simulink model "PuntoEquilibrio"  (R2015a)
settings: Solver=ode45  StartTime=0.0  StopTime=50  RelTol=1e-3
values from neighbouring files (symbols this model uses):
  b = 2.64e-4    (= 0.000264)    [ParametrosQuadcoptero.m]
  d = 7.5e-7    (= 7.5e-07)    [ParametrosQuadcoptero.m]
  g = 9.81    [ParametrosQuadcoptero.m]
  Ix = 0.033    [ParametrosQuadcoptero.m]
  Iy = 0.033    [ParametrosQuadcoptero.m]
  Iz = 0.066    [ParametrosQuadcoptero.m]
  L = 0.5    [ParametrosQuadcoptero.m]
  m = 4    [ParametrosQuadcoptero.m]
  sys = ss(A,B,C,D,Ts)    [ModeloVariablesEstado.m]
  Ts = 0.05    [ModeloVariablesEstado.m]
  x10_0 = 0    [CondicionesIniciales.m]
  x11_0 = 0    [CondicionesIniciales.m]
  x12_0 = 0    [CondicionesIniciales.m]
  x1_0 = 0    [CondicionesIniciales.m]
  x2_0 = 0    [CondicionesIniciales.m]
  x3_0 = 0    [CondicionesIniciales.m]
  x4_0 = 0    [CondicionesIniciales.m]
  x5_0 = 10    [CondicionesIniciales.m]
  x6_0 = 0    [CondicionesIniciales.m]
  x7_0 = 0    [CondicionesIniciales.m]
  x8_0 = 0    [CondicionesIniciales.m]
  x9_0 = 0    [CondicionesIniciales.m]
libraries: mpclib x1
settings Model: Creator=Dell  LastModifiedBy=Dell

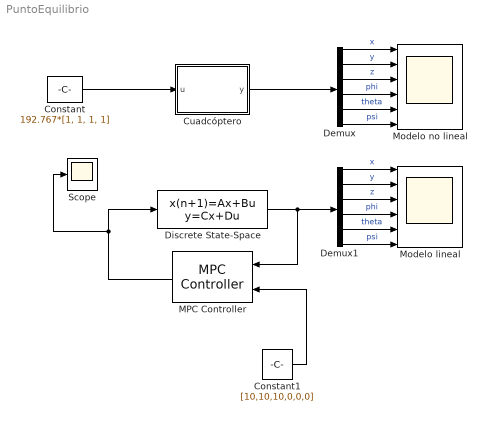
== system PuntoEquilibrio ==
  Constant : Constant  Value=192.767*[1, 1, 1, 1]
  Constant1 : Constant  Value=[10,10,10,0,0,0]  SampleTime=Ts
  Cuadcóptero : Subsystem
  Demux : Demux  Outputs=6
  Demux1 : Demux  Outputs=6
  Discrete State-Space : DiscreteStateSpace  A=sys.A  B=sys.B  C=sys.C  D=sys.D  X0=[x1_0,x2_0,x3_0,x4_0,x5_0,x6_0,x7_0,x8_0,x9_0,x10_0,x11_0,x12_0]  SampleTime=Ts
  MPC Controller : mpclib/MPC Controller  SCDEnableBlockLinearizationSpecification=on  mpcobj=MPC1  is_multiple=0  enable_value=0  n_mv=4  n_mo=6  n_md=0  n_ts=0.05  is_designfromscratch=0  return_u0=off  ref_from_ws=off  ref_signal_name=[]  ref_preview=off  md_from_ws=off  md_signal_name=[]  md_preview=off  from_project=off  project_file=MPCtask.mat  md_inport=off  mv_inport=off  cost_outport=off  return_sequence=off  return_qpstatus=off  return_state=off  state_inport=off  lims_inport=off  ywt_inport=off  uwt_inport=off  duwt_inport=off  rhoeps_inport=off  uref_inport=off  BlockDataType=double  SampleTimeInherited=off  switch_inport=off
  Modelo lineal : Scope  NumInputPorts=6
      settings: TickLabels=on  YMin=-5~-5~-5~-5~-5~-5  YMax=5~5~5~5~5~5
  Modelo no lineal : Scope  NumInputPorts=6
      settings: TickLabels=on  YMin=-5~-5~-5~-5~-5~-5  YMax=5~5~5~5~5~5
  Scope : Scope
      settings: SaveName=ScopeData2
  wires:
  Constant/1 -> Cuadcóptero/1(u)
  Cuadcóptero/1(y) -> Demux/1
  Demux/1 -> Modelo no lineal/1  "x"
  Demux/2 -> Modelo no lineal/2  "y"
  Demux/3 -> Modelo no lineal/3  "z"
  Demux/4 -> Modelo no lineal/4  "phi"
  Demux/5 -> Modelo no lineal/5  "theta"
  Demux/6 -> Modelo no lineal/6  "psi"
  Discrete State-Space/1 -> MPC Controller/1, Demux1/1
  Demux1/1 -> Modelo lineal/1  "x"
  Demux1/2 -> Modelo lineal/2  "y"
  Demux1/3 -> Modelo lineal/3  "z"
  Demux1/4 -> Modelo lineal/4  "phi"
  Demux1/5 -> Modelo lineal/5  "theta"
  Demux1/6 -> Modelo lineal/6  "psi"
  MPC Controller/1 -> Scope/1, Discrete State-Space/1
  Constant1/1 -> MPC Controller/2

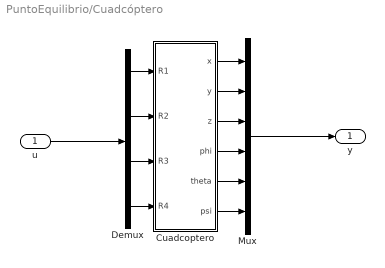
== system PuntoEquilibrio/Cuadcóptero ==
  u : Inport
  Cuadcoptero : Subsystem
  Demux : Demux
  Mux : Mux  Inputs=6
  y : Outport
  wires:
  Cuadcoptero/5(theta) -> Mux/5
  Cuadcoptero/1(x) -> Mux/1
  Cuadcoptero/3(z) -> Mux/3
  Cuadcoptero/2(y) -> Mux/2
  Mux/1 -> y/1
  Demux/4 -> Cuadcoptero/4(R4)
  Demux/1 -> Cuadcoptero/1(R1)
  Demux/2 -> Cuadcoptero/2(R2)
  Demux/3 -> Cuadcoptero/3(R3)
  Cuadcoptero/4(phi) -> Mux/4
  Cuadcoptero/6(psi) -> Mux/6
  u/1 -> Demux/1

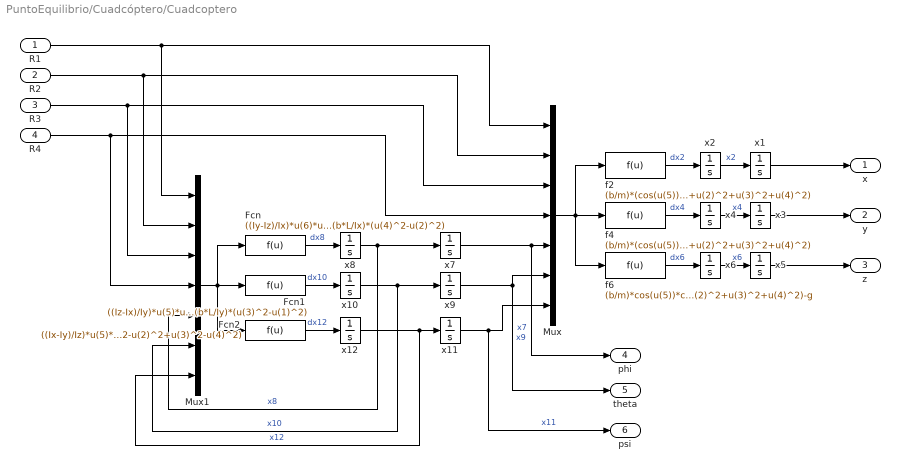
== system PuntoEquilibrio/Cuadcóptero/Cuadcoptero ==
  R1 : Inport
  R2 : Inport  Port=2
  R3 : Inport  Port=3
  R4 : Inport  Port=4
  Fcn : Fcn  Expr=((Iy-Iz)/Ix)*u(6)*u(7)+(b*L/Ix)*(u(4)^2-u(2)^2)
  Fcn1 : Fcn  Expr=((Iz-Ix)/Iy)*u(5)*u(7)+(b*L/Iy)*(u(3)^2-u(1)^2)
  Fcn2 : Fcn  Expr=((Ix-Iy)/Iz)*u(5)*u(6)+(d/Iz)*(u(1)^2-u(2)^2+u(3)^2-u(4)^2)
  Mux : Mux  Inputs=7
  Mux1 : Mux  Inputs=7
  f2 : Fcn  Expr=(b/m)*(cos(u(5))*sin(u(6))*cos(u(7))+sin(u(5))*sin(u(7)))*(u(1)^2+u(2)^2+u(3)^2+u(4)^2)
  f4 : Fcn  Expr=(b/m)*(cos(u(5))*sin(u(6))*sin(u(7))-sin(u(5))*cos(u(7)))*(u(1)^2+u(2)^2+u(3)^2+u(4)^2)
  f6 : Fcn  Expr=(b/m)*cos(u(5))*cos(u(6))*(u(1)^2+u(2)^2+u(3)^2+u(4)^2)-g
  x1 : Integrator  InitialCondition=x1_0
  x10 : Integrator  InitialCondition=x10_0
  x11 : Integrator  InitialCondition=x11_0
  x12 : Integrator  InitialCondition=x12_0
  x2 : Integrator  InitialCondition=x2_0
  x3 : Integrator  InitialCondition=x3_0
  x4 : Integrator  InitialCondition=x4_0
  x5 : Integrator  InitialCondition=x5_0
  x6 : Integrator  InitialCondition=x6_0
  x7 : Integrator  InitialCondition=x7_0
  x8 : Integrator  InitialCondition=x8_0
  x9 : Integrator  InitialCondition=x9_0
  x : Outport
  y : Outport  Port=2
  z : Outport  Port=3
  phi : Outport  Port=4
  theta : Outport  Port=5
  psi : Outport  Port=6
  wires:
  x12/1 -> x11/1, Mux1/7  "x12"
  x6/1 -> x5/1  "x6"
  x2/1 -> x1/1  "x2"
  x8/1 -> Mux1/5, x7/1  "x8"
  x4/1 -> x3/1  "x4"
  x10/1 -> x9/1, Mux1/6  "x10"
  Fcn1/1 -> x10/1  "dx10"
  x7/1 -> phi/1, Mux/5  "x7"
  x5/1 -> z/1
  f2/1 -> x2/1  "dx2"
  x1/1 -> x/1
  x11/1 -> psi/1, Mux/7  "x11"
  f4/1 -> x4/1  "dx4"
  R3/1 -> Mux1/3, Mux/3
  R4/1 -> Mux1/4, Mux/4
  R2/1 -> Mux1/2, Mux/2
  f6/1 -> x6/1  "dx6"
  R1/1 -> Mux1/1, Mux/1
  x9/1 -> theta/1, Mux/6  "x9"
  Mux/1 -> f6/1, f2/1, f4/1
  Fcn/1 -> x8/1  "dx8"
  Mux1/1 -> Fcn1/1, Fcn/1, Fcn2/1
  Fcn2/1 -> x12/1  "dx12"
  x3/1 -> y/1
